simulink library "SunTorqueC"  (R2014b)
settings: Solver=ode45  StartTime=0.0  StopTime=10.0  RelTol=1e-3
undefined symbols (not defined in the file or in its folder): ConfParam
libraries: Eclipse x1
settings Model: Creator=Hp  LastModifiedBy=Hp

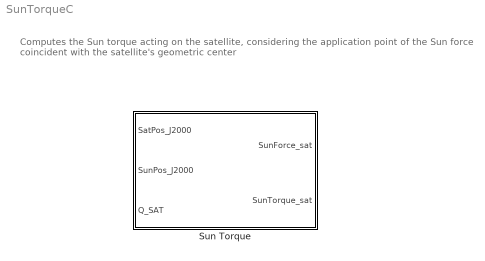
== system SunTorqueC ==
  note: Computes the Sun torque acting on the satellite,
      | considering the application point of the Sun force
      | coincident with the satellite's geometric center
  Sun Torque : Subsystem

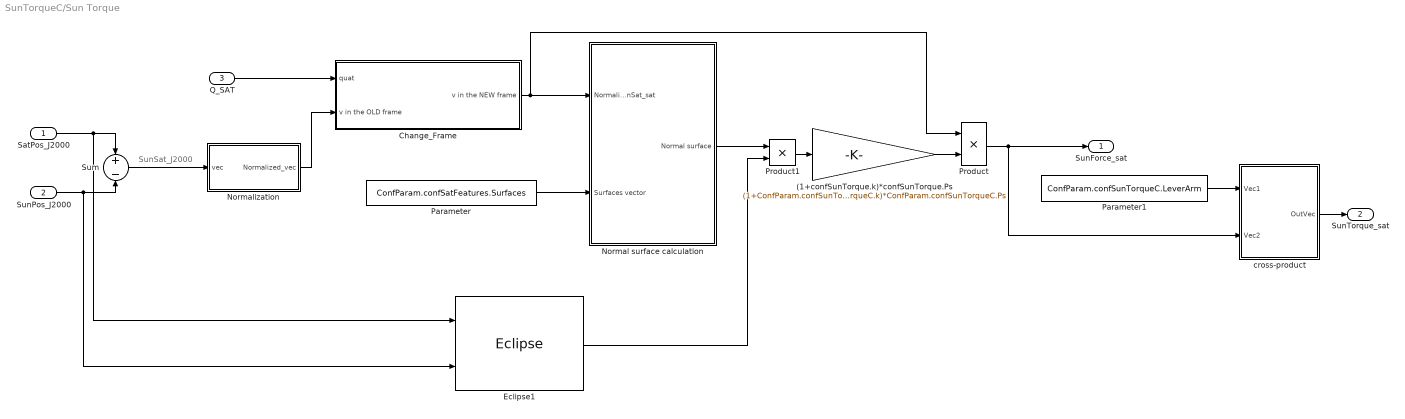
== system SunTorqueC/Sun Torque ==
  note: SunSat_J2000
  SatPos_J2000 : Inport
  SunPos_J2000 : Inport  Port=2
  Q_SAT : Inport  Port=3
  (1+confSunTorque.k)*confSunTorque.Ps : Gain  Gain=(1+ConfParam.confSunTorqueC.k)*ConfParam.confSunTorqueC.Ps
  Change_Frame : Subsystem
  Eclipse1 : Eclipse/Eclipse
  Normal surface calculation : Subsystem
  Normalization : Subsystem
  Parameter : Constant  Value=ConfParam.confSatFeatures.Surfaces
  Parameter1 : Constant  Value=ConfParam.confSunTorqueC.LeverArm
  Product : Product
  Product1 : Product
  Sum : Sum  Inputs=+-
  cross-product : Subsystem
  SunForce_sat : Outport
  SunTorque_sat : Outport  Port=2
  wires:
  Product1/1 -> (1+confSunTorque.k)*confSunTorque.Ps/1
  Normal surface calculation/1(Normal surface) -> Product1/1
  Eclipse1/1 -> Product1/2
  cross-product/1(OutVec) -> SunTorque_sat/1
  Parameter1/1 -> cross-product/1(Vec1)
  Product/1 -> SunForce_sat/1, cross-product/2(Vec2)
  (1+confSunTorque.k)*confSunTorque.Ps/1 -> Product/2
  Parameter/1 -> Normal surface calculation/2(Surfaces vector)
  Change_Frame/1(v in the NEW frame) -> Normal surface calculation/1("Normalized SunSat_sat "), Product/1
  Normalization/1(Normalized_vec) -> Change_Frame/2(v in the OLD frame)
  Q_SAT/1 -> Change_Frame/1(quat)
  Sum/1 -> Normalization/1(vec)
  SunPos_J2000/1 -> Eclipse1/2, Sum/2
  SatPos_J2000/1 -> Eclipse1/1, Sum/1

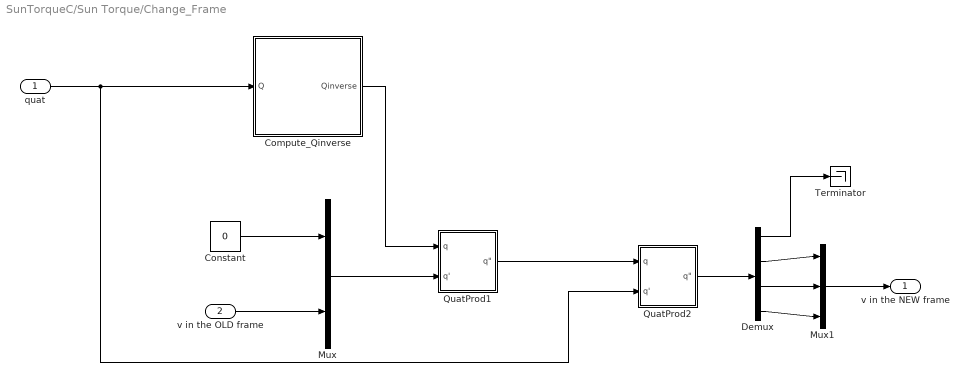
== system SunTorqueC/Sun Torque/Change_Frame ==
  quat : Inport
  v in the OLD frame : Inport  Port=2
  Compute_Qinverse : Subsystem
  Constant : Constant  Value=0
  Demux : Demux
  Mux : Mux  Inputs=2
  Mux1 : Mux  Inputs=3
  QuatProd1 : Subsystem  TreatAsAtomicUnit=on
      settings: RTWFcnNameOpts=Use subsystem name  RTWFileNameOpts=Use subsystem name
  QuatProd2 : Subsystem  TreatAsAtomicUnit=on
      settings: RTWFcnNameOpts=Use subsystem name  RTWFileNameOpts=Use subsystem name
  Terminator : Terminator
  v in the NEW frame : Outport
  wires:
  quat/1 -> QuatProd2/2(q'), Compute_Qinverse/1(Q)
  Demux/1 -> Terminator/1
  v in the OLD frame/1 -> Mux/2
  Mux/1 -> QuatProd1/2(q')
  Constant/1 -> Mux/1
  Compute_Qinverse/1(Qinverse) -> QuatProd1/1(q)
  Mux1/1 -> v in the NEW frame/1
  Demux/2 -> Mux1/1
  Demux/3 -> Mux1/2
  Demux/4 -> Mux1/3
  QuatProd1/1("q\"") -> QuatProd2/1(q)
  QuatProd2/1("q\"") -> Demux/1

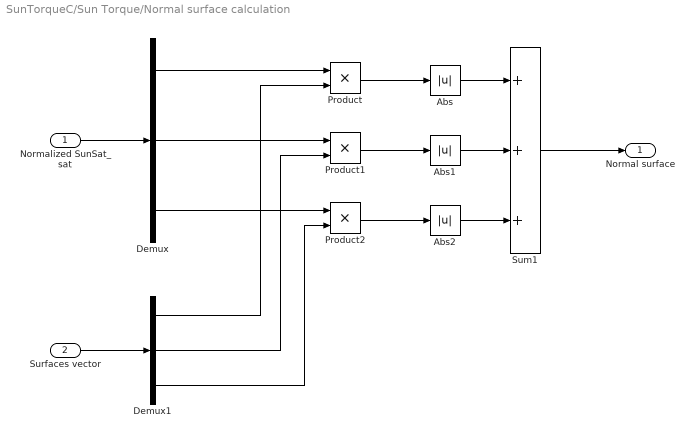
== system SunTorqueC/Sun Torque/Normal surface calculation ==
  "Normalized SunSat_sat " : Inport
  Surfaces vector : Inport  Port=2
  Abs : Abs
  Abs1 : Abs
  Abs2 : Abs
  Demux : Demux  Outputs=3
  Demux1 : Demux  Outputs=3
  Product : Product
  Product1 : Product
  Product2 : Product
  Sum1 : Sum  Inputs=+++
  Normal surface : Outport
  wires:
  Demux/1 -> Product/1
  Abs2/1 -> Sum1/3
  Product1/1 -> Abs1/1
  Demux1/3 -> Product2/2
  Demux1/2 -> Product1/2
  Surfaces vector/1 -> Demux1/1
  Product2/1 -> Abs2/1
  Product/1 -> Abs/1
  Abs1/1 -> Sum1/2
  "Normalized SunSat_sat "/1 -> Demux/1
  Sum1/1 -> Normal surface/1
  Demux1/1 -> Product/2
  Demux/2 -> Product1/1
  Demux/3 -> Product2/1
  Abs/1 -> Sum1/1

== system SunTorqueC/Sun Torque/Normalization ==
  vec : Inport
  ComputeNorm3D : Subsystem
  Division vector/scalar : Subsystem
  Normalized_vec : Outport
  wires:
  vec/1 -> Division vector/scalar/1(vec), ComputeNorm3D/1(vector3D)
  Division vector/scalar/1(result_vec) -> Normalized_vec/1
  ComputeNorm3D/1(Norm) -> Division vector/scalar/2(scalar)

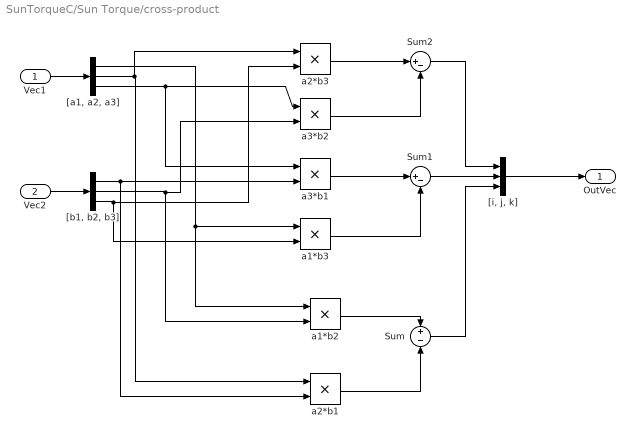
== system SunTorqueC/Sun Torque/cross-product ==
  Vec1 : Inport
  Vec2 : Inport  Port=2
  Sum : Sum  Inputs=+-
  Sum1 : Sum  Inputs=|+-
  Sum2 : Sum  Inputs=|+-
  "[a1, a2, a3]" : Demux  Outputs=3
  "[b1, b2, b3]" : Demux  Outputs=3
  "[i, j, k]" : Mux  Inputs=3
  a1*b2 : Product
  a1*b3 : Product
  a2*b1 : Product
  a2*b3 : Product
  a3*b1 : Product
  a3*b2 : Product
  OutVec : Outport
  wires:
  Sum1/1 -> "[i, j, k]"/2
  Sum2/1 -> "[i, j, k]"/1
  Sum/1 -> "[i, j, k]"/3
  a3*b2/1 -> Sum2/2
  "[i, j, k]"/1 -> OutVec/1
  a1*b3/1 -> Sum1/2
  "[b1, b2, b3]"/3 -> a1*b3/2, a2*b3/2
  a2*b3/1 -> Sum2/1
  "[a1, a2, a3]"/3 -> a3*b2/1, a3*b1/1
  a3*b1/1 -> Sum1/1
  a1*b2/1 -> Sum/1
  "[b1, b2, b3]"/2 -> a1*b2/2, a3*b2/2
  Vec1/1 -> "[a1, a2, a3]"/1
  "[a1, a2, a3]"/1 -> a1*b2/1, a1*b3/1
  Vec2/1 -> "[b1, b2, b3]"/1
  "[a1, a2, a3]"/2 -> a2*b1/1, a2*b3/1
  "[b1, b2, b3]"/1 -> a2*b1/2, a3*b1/2
  a2*b1/1 -> Sum/2

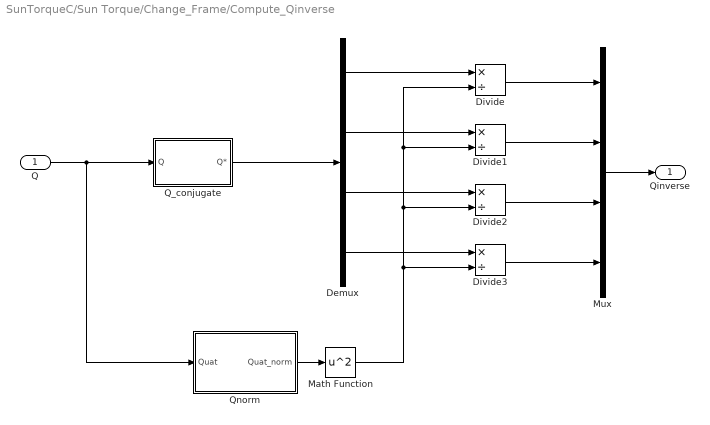
== system SunTorqueC/Sun Torque/Change_Frame/Compute_Qinverse ==
  Q : Inport
  Demux : Demux
  Divide{,1..3} (4 alike) : Product  Inputs=*/
  Math Function : Math  Operator=square  SaturateOnIntegerOverflow=on
  Mux : Mux
  Q_conjugate : Subsystem
  Qnorm : Subsystem
  Qinverse : Outport
  wires:
  Mux/1 -> Qinverse/1
  Demux/2 -> Divide1/1
  Divide2/1 -> Mux/3
  Q_conjugate/1(Q*) -> Demux/1
  Divide/1 -> Mux/1
  Divide1/1 -> Mux/2
  Divide3/1 -> Mux/4
  Q/1 -> Q_conjugate/1(Q), Qnorm/1(Quat)
  Demux/4 -> Divide3/1
  Qnorm/1(Quat_norm) -> Math Function/1
  Demux/1 -> Divide/1
  Demux/3 -> Divide2/1
  Math Function/1 -> Divide/2, Divide1/2, Divide2/2, Divide3/2

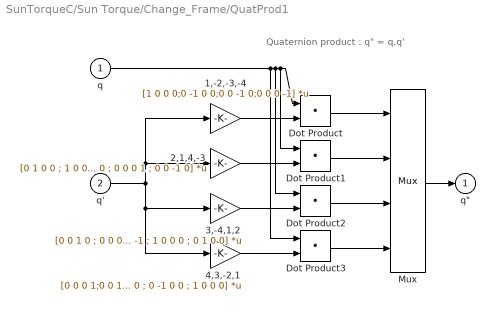
== system SunTorqueC/Sun Torque/Change_Frame/QuatProd1 ==
  note: Quaternion product : q" = q.q'
  q : Inport  OutDataTypeStr=double  PortDimensions=4
  q' : Inport  Port=2  OutDataTypeStr=double  PortDimensions=4
  1,-2,-3,-4 : Gain  Gain=[1 0 0 0;0 -1 0 0;0 0 -1 0;0 0 0 -1]  Multiplication=Matrix(K*u) (u vector)  SaturateOnIntegerOverflow=on  OutDataTypeStr=Inherit: Same as input  ParamDataTypeStr=Inherit: Same as input
  2,1,4,-3 : Gain  Gain=[0 1 0 0 ; 1 0 0 0 ; 0 0 0 1 ; 0 0 -1 0]  Multiplication=Matrix(K*u) (u vector)  SaturateOnIntegerOverflow=on  OutDataTypeStr=Inherit: Same as input  ParamDataTypeStr=Inherit: Same as input
  3,-4,1,2 : Gain  Gain=[0 0 1 0 ; 0 0 0 -1 ; 1 0 0 0 ; 0 1 0 0]  Multiplication=Matrix(K*u) (u vector)  SaturateOnIntegerOverflow=on  OutDataTypeStr=Inherit: Same as input  ParamDataTypeStr=Inherit: Same as input
  4,3,-2,1 : Gain  Gain=[0 0 0 1;0 0 1 0 ; 0 -1 0 0 ; 1 0 0 0]  Multiplication=Matrix(K*u) (u vector)  SaturateOnIntegerOverflow=on  OutDataTypeStr=Inherit: Same as input  ParamDataTypeStr=Inherit: Same as input
  Dot Product{,1..3} (4 alike) : DotProduct  InputSameDT=on  OutDataTypeStr=Inherit: Inherit via internal rule
  Mux : Mux
  "q\"" : Outport  OutDataTypeStr=double  PortDimensions=4  InitialOutput=0
  wires:
  q'/1 -> 3,-4,1,2/1, 4,3,-2,1/1, 1,-2,-3,-4/1, 2,1,4,-3/1
  1,-2,-3,-4/1 -> Dot Product/2
  2,1,4,-3/1 -> Dot Product1/2
  3,-4,1,2/1 -> Dot Product2/2
  4,3,-2,1/1 -> Dot Product3/2
  q/1 -> Dot Product/1, Dot Product1/1, Dot Product2/1, Dot Product3/1
  Dot Product/1 -> Mux/1
  Dot Product1/1 -> Mux/2
  Dot Product2/1 -> Mux/3
  Dot Product3/1 -> Mux/4
  Mux/1 -> "q\""/1

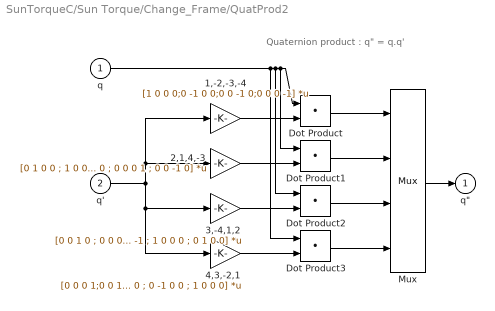
== system SunTorqueC/Sun Torque/Change_Frame/QuatProd2 ==
  note: Quaternion product : q" = q.q'
  q : Inport  OutDataTypeStr=double  PortDimensions=4
  q' : Inport  Port=2  OutDataTypeStr=double  PortDimensions=4
  1,-2,-3,-4 : Gain  Gain=[1 0 0 0;0 -1 0 0;0 0 -1 0;0 0 0 -1]  Multiplication=Matrix(K*u) (u vector)  SaturateOnIntegerOverflow=on  OutDataTypeStr=Inherit: Same as input  ParamDataTypeStr=Inherit: Same as input
  2,1,4,-3 : Gain  Gain=[0 1 0 0 ; 1 0 0 0 ; 0 0 0 1 ; 0 0 -1 0]  Multiplication=Matrix(K*u) (u vector)  SaturateOnIntegerOverflow=on  OutDataTypeStr=Inherit: Same as input  ParamDataTypeStr=Inherit: Same as input
  3,-4,1,2 : Gain  Gain=[0 0 1 0 ; 0 0 0 -1 ; 1 0 0 0 ; 0 1 0 0]  Multiplication=Matrix(K*u) (u vector)  SaturateOnIntegerOverflow=on  OutDataTypeStr=Inherit: Same as input  ParamDataTypeStr=Inherit: Same as input
  4,3,-2,1 : Gain  Gain=[0 0 0 1;0 0 1 0 ; 0 -1 0 0 ; 1 0 0 0]  Multiplication=Matrix(K*u) (u vector)  SaturateOnIntegerOverflow=on  OutDataTypeStr=Inherit: Same as input  ParamDataTypeStr=Inherit: Same as input
  Dot Product{,1..3} (4 alike) : DotProduct  InputSameDT=on  OutDataTypeStr=Inherit: Inherit via internal rule
  Mux : Mux
  "q\"" : Outport  OutDataTypeStr=double  PortDimensions=4  InitialOutput=0
  wires:
  q'/1 -> 3,-4,1,2/1, 4,3,-2,1/1, 1,-2,-3,-4/1, 2,1,4,-3/1
  1,-2,-3,-4/1 -> Dot Product/2
  2,1,4,-3/1 -> Dot Product1/2
  3,-4,1,2/1 -> Dot Product2/2
  4,3,-2,1/1 -> Dot Product3/2
  q/1 -> Dot Product/1, Dot Product1/1, Dot Product2/1, Dot Product3/1
  Dot Product/1 -> Mux/1
  Dot Product1/1 -> Mux/2
  Dot Product2/1 -> Mux/3
  Dot Product3/1 -> Mux/4
  Mux/1 -> "q\""/1

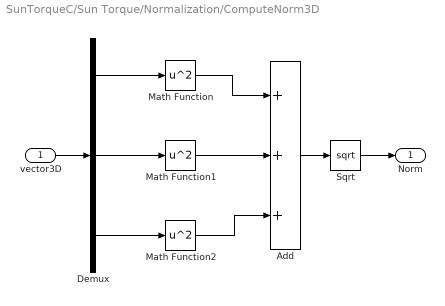
== system SunTorqueC/Sun Torque/Normalization/ComputeNorm3D ==
  vector3D : Inport
  Add : Sum  Inputs=+++
  Demux : Demux  Outputs=3
  Math Function : Math  Operator=square  SaturateOnIntegerOverflow=on
  Math Function1 : Math  Operator=square  SaturateOnIntegerOverflow=on
  Math Function2 : Math  Operator=square  SaturateOnIntegerOverflow=on
  Sqrt : Sqrt  SaturateOnIntegerOverflow=on
  Norm : Outport
  wires:
  vector3D/1 -> Demux/1
  Sqrt/1 -> Norm/1
  Add/1 -> Sqrt/1
  Math Function1/1 -> Add/2
  Math Function2/1 -> Add/3
  Demux/1 -> Math Function/1
  Math Function/1 -> Add/1
  Demux/3 -> Math Function2/1
  Demux/2 -> Math Function1/1

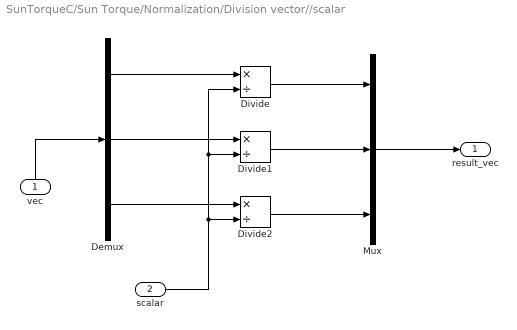
== system SunTorqueC/Sun Torque/Normalization/Division vector//scalar ==
  vec : Inport
  scalar : Inport  Port=2
  Demux : Demux  Outputs=3
  Divide : Product  Inputs=*/
  Divide1 : Product  Inputs=*/
  Divide2 : Product  Inputs=*/
  Mux : Mux  Inputs=3
  result_vec : Outport
  wires:
  Divide/1 -> Mux/1
  Mux/1 -> result_vec/1
  scalar/1 -> Divide1/2, Divide/2, Divide2/2
  Demux/3 -> Divide2/1
  Divide2/1 -> Mux/3
  Divide1/1 -> Mux/2
  Demux/1 -> Divide/1
  Demux/2 -> Divide1/1
  vec/1 -> Demux/1

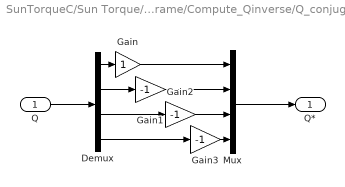
== system SunTorqueC/Sun Torque/Change_Frame/Compute_Qinverse/Q_conjugate ==
  Q : Inport
  Demux : Demux
  Gain : Gain
  Gain1 : Gain  Gain=-1
  Gain2 : Gain  Gain=-1
  Gain3 : Gain  Gain=-1
  Mux : Mux
  Q* : Outport
  wires:
  Gain3/1 -> Mux/4
  Q/1 -> Demux/1
  Gain2/1 -> Mux/3
  Demux/2 -> Gain1/1
  Demux/3 -> Gain2/1
  Gain1/1 -> Mux/2
  Demux/4 -> Gain3/1
  Mux/1 -> Q*/1
  Gain/1 -> Mux/1
  Demux/1 -> Gain/1

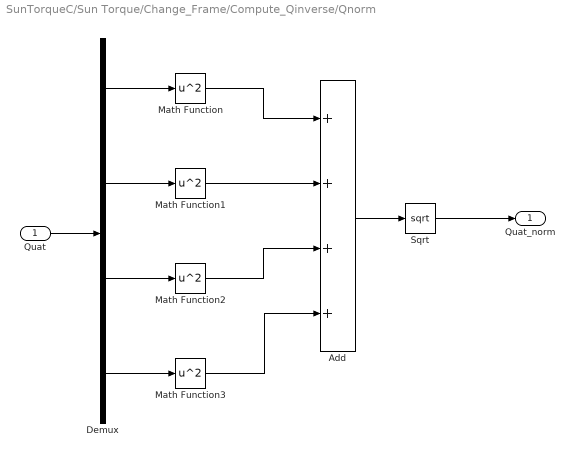
== system SunTorqueC/Sun Torque/Change_Frame/Compute_Qinverse/Qnorm ==
  Quat : Inport
  Add : Sum  Inputs=++++
  Demux : Demux
  Math Function{,1..3} (4 alike) : Math  Operator=square  SaturateOnIntegerOverflow=on
  Sqrt : Sqrt  SaturateOnIntegerOverflow=on
  Quat_norm : Outport
  wires:
  Quat/1 -> Demux/1
  Demux/2 -> Math Function1/1
  Sqrt/1 -> Quat_norm/1
  Demux/4 -> Math Function3/1
  Demux/1 -> Math Function/1
  Demux/3 -> Math Function2/1
  Math Function1/1 -> Add/2
  Math Function3/1 -> Add/4
  Add/1 -> Sqrt/1
  Math Function/1 -> Add/1
  Math Function2/1 -> Add/3
